simulink model "Stone"  (Simulink 7.6)
settings: Solver=ode5  StartTime=0.0  StopTime=10.0  FixedStep=0.01  RelTol=1e-3
libraries: simulink x1
settings Model: Creator=Podolsky  LastModifiedBy=Podolsky
settings DataIOCC: SignalLoggingName=sigsOut
settings DebuggingCC: SaveWithParameterizedLinksMsg=none  SignalResolutionControl=TryResolveAllWithWarning  SolverPrmCheckMsg=none  MultiTaskDSMMsg=warning  MultiTaskCondExecSysMsg=none  StrictBusMsg=None
settings HardwareCC: TargetUnknown=on
settings RTWCC: IncludeERTFirstTime=on

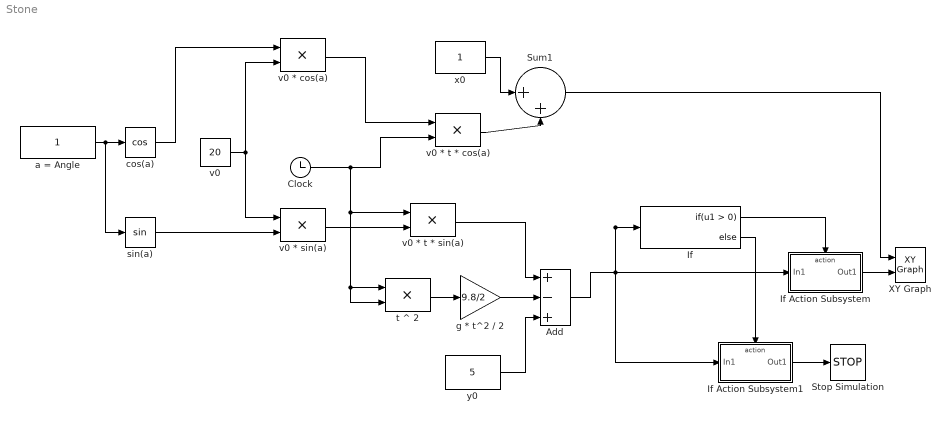
== system Stone ==
  Add : Sum  Inputs=+-+
  Clock : Clock
      settings: Decimation=5
  If : If
  If Action Subsystem : Subsystem  TreatAsAtomicUnit=on
  If Action Subsystem1 : Subsystem  TreatAsAtomicUnit=on
  Stop Simulation : Stop
  Sum1 : Sum  Inputs=|++
  XY Graph : simulink/Sinks/XY Graph  SystemSampleTime=-1  xmin=0  xmax=42  ymin=0  ymax=42  st=-1
  a = Angle : Constant
  cos(a) : Trigonometry  Operator=cos
  g * t^2 / 2 : Gain  Gain=9.8/2  SaturateOnIntegerOverflow=on  OutDataTypeStr=Inherit: Same as input  ParamDataTypeStr=Inherit: Same as input
  sin(a) : Trigonometry
  t ^ 2 : Product  SaturateOnIntegerOverflow=on  OutDataTypeStr=Inherit: Same as first input
  v0 : Constant  Value=20
  v0 * cos(a) : Product  SaturateOnIntegerOverflow=on  OutDataTypeStr=Inherit: Same as first input
  v0 * sin(a) : Product  SaturateOnIntegerOverflow=on  OutDataTypeStr=Inherit: Same as first input
  v0 * t * cos(a) : Product  SaturateOnIntegerOverflow=on  OutDataTypeStr=Inherit: Same as first input
  v0 * t * sin(a) : Product  SaturateOnIntegerOverflow=on  OutDataTypeStr=Inherit: Same as first input
  x0 : Constant
  y0 : Constant  Value=5
  wires:
  a = Angle/1 -> cos(a)/1, sin(a)/1
  t ^ 2/1 -> g * t^2 / 2/1
  Clock/1 -> v0 * t * sin(a)/1, t ^ 2/1, t ^ 2/2, v0 * t * cos(a)/2
  Add/1 -> If/1, If Action Subsystem/1(In1), If Action Subsystem1/1(In1)
  If/1 -> If Action Subsystem/Action
  If Action Subsystem/1(Out1) -> XY Graph/2
  If/2 -> If Action Subsystem1/Action
  If Action Subsystem1/1(Out1) -> Stop Simulation/1
  Sum1/1 -> XY Graph/1
  x0/1 -> Sum1/1
  v0 * t * cos(a)/1 -> Sum1/2
  sin(a)/1 -> v0 * sin(a)/2
  cos(a)/1 -> v0 * cos(a)/1
  v0 * sin(a)/1 -> v0 * t * sin(a)/2
  v0 * cos(a)/1 -> v0 * t * cos(a)/1
  g * t^2 / 2/1 -> Add/2
  v0 * t * sin(a)/1 -> Add/1
  y0/1 -> Add/3
  v0/1 -> v0 * cos(a)/2, v0 * sin(a)/1

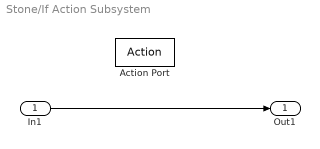
== system Stone/If Action Subsystem ==
  In1 : Inport
  Action Port : ActionPort  ActionType=then
  Out1 : Outport
  wires:
  In1/1 -> Out1/1

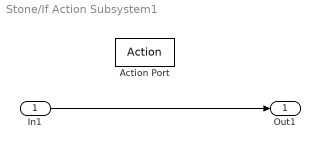
== system Stone/If Action Subsystem1 ==
  In1 : Inport
  Action Port : ActionPort  ActionType=else
  Out1 : Outport
  wires:
  In1/1 -> Out1/1
